simulink library "INT_CoETS_TSEACo"  (R2016b)
settings: Solver=VariableStepAuto  StartTime=0.0  StopTime=10.0  RelTol=1e-3
settings Model: Creator=xuxingpei  LastModifiedBy=xuxingpei

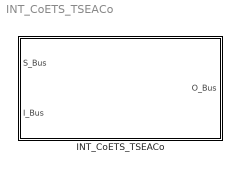
== system INT_CoETS_TSEACo ==
  INT_CoETS_TSEACo : Subsystem

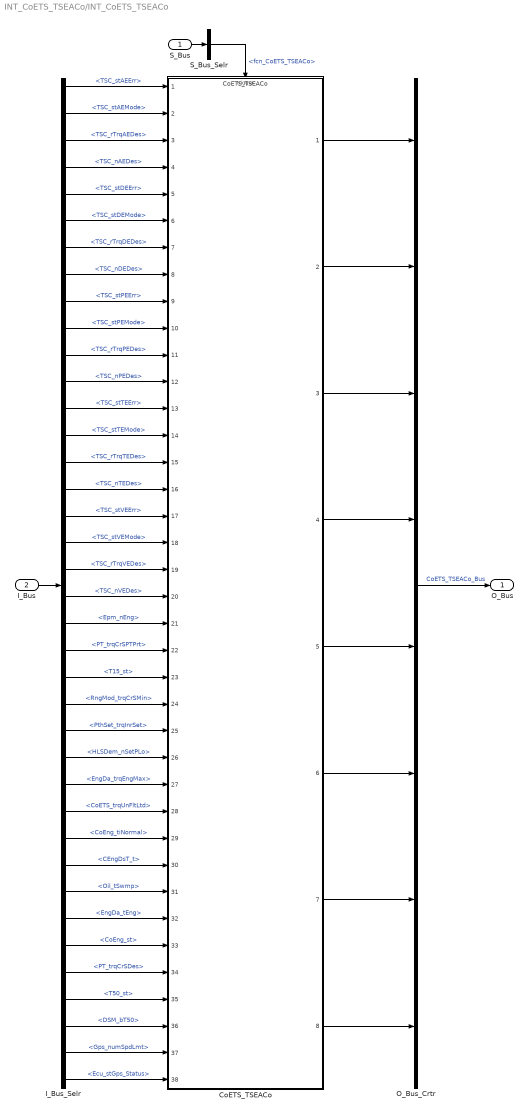
== system INT_CoETS_TSEACo/INT_CoETS_TSEACo ==
  S_Bus : Inport
  I_Bus : Inport  Port=2
  CoETS_TSEACo : ModelReference  ModelNameDialog=CoETS_TSEACo  SimulationMode=Normal  ModelReferenceVersion=1.404  TriggerPortName=function  TriggerPortTriggerType=function-call  TriggerPortStatesWhenEnabling=held
  I_Bus_Selr : BusSelector  OutputSignals=TSC_stAEErr,TSC_stAEMode,TSC_rTrqAEDes,TSC_nAEDes,TSC_stDEErr,TSC_stDEMode,TSC_rTrqDEDes,TSC_nDEDes,TSC_stPEErr,TSC_stPEMode,TSC_rTrqPEDes,TSC_nPEDes,TSC_stTEErr,TSC_stTEMode,TSC_rTrqTEDes,TSC_nTEDes,TSC_stVEErr,TSC_stVEMode,TSC_rTrqVEDes,TSC_nVEDes,Epm_nEng,PT_trqCrSPTPrt,T15_st,RngMod_trqCrSMin,PthSet_trqInrSet,HLSDem_nSetPLo,EngDa_trqEngMax,CoETS_trqUnFltLtd,CoEng_tiNormal,CEngDsT_t,Oil_tSwmp,EngDa_tEng,CoEng_st,PT_trqCrSDes,T50_st,DSM_bT50,Gps_numSpdLmt,Ecu_stGps_Status
  O_Bus_Crtr : BusCreator  Inputs=8
  S_Bus_Selr : BusSelector  OutputSignals=fcn_CoETS_TSEACo
  O_Bus : Outport
  wires:
  S_Bus_Selr/1 -> CoETS_TSEACo/Trigger  "<fcn_CoETS_TSEACo>"
  S_Bus/1 -> S_Bus_Selr/1
  I_Bus/1 -> I_Bus_Selr/1
  I_Bus_Selr/1 -> CoETS_TSEACo/1  "<TSC_stAEErr>"
  I_Bus_Selr/2 -> CoETS_TSEACo/2  "<TSC_stAEMode>"
  I_Bus_Selr/3 -> CoETS_TSEACo/3  "<TSC_rTrqAEDes>"
  I_Bus_Selr/4 -> CoETS_TSEACo/4  "<TSC_nAEDes>"
  I_Bus_Selr/5 -> CoETS_TSEACo/5  "<TSC_stDEErr>"
  I_Bus_Selr/6 -> CoETS_TSEACo/6  "<TSC_stDEMode>"
  I_Bus_Selr/7 -> CoETS_TSEACo/7  "<TSC_rTrqDEDes>"
  I_Bus_Selr/8 -> CoETS_TSEACo/8  "<TSC_nDEDes>"
  I_Bus_Selr/9 -> CoETS_TSEACo/9  "<TSC_stPEErr>"
  I_Bus_Selr/10 -> CoETS_TSEACo/10  "<TSC_stPEMode>"
  I_Bus_Selr/11 -> CoETS_TSEACo/11  "<TSC_rTrqPEDes>"
  I_Bus_Selr/12 -> CoETS_TSEACo/12  "<TSC_nPEDes>"
  I_Bus_Selr/13 -> CoETS_TSEACo/13  "<TSC_stTEErr>"
  I_Bus_Selr/14 -> CoETS_TSEACo/14  "<TSC_stTEMode>"
  I_Bus_Selr/15 -> CoETS_TSEACo/15  "<TSC_rTrqTEDes>"
  I_Bus_Selr/16 -> CoETS_TSEACo/16  "<TSC_nTEDes>"
  I_Bus_Selr/17 -> CoETS_TSEACo/17  "<TSC_stVEErr>"
  I_Bus_Selr/18 -> CoETS_TSEACo/18  "<TSC_stVEMode>"
  I_Bus_Selr/19 -> CoETS_TSEACo/19  "<TSC_rTrqVEDes>"
  I_Bus_Selr/20 -> CoETS_TSEACo/20  "<TSC_nVEDes>"
  I_Bus_Selr/21 -> CoETS_TSEACo/21  "<Epm_nEng>"
  I_Bus_Selr/22 -> CoETS_TSEACo/22  "<PT_trqCrSPTPrt>"
  I_Bus_Selr/23 -> CoETS_TSEACo/23  "<T15_st>"
  I_Bus_Selr/24 -> CoETS_TSEACo/24  "<RngMod_trqCrSMin>"
  I_Bus_Selr/25 -> CoETS_TSEACo/25  "<PthSet_trqInrSet>"
  I_Bus_Selr/26 -> CoETS_TSEACo/26  "<HLSDem_nSetPLo>"
  I_Bus_Selr/27 -> CoETS_TSEACo/27  "<EngDa_trqEngMax>"
  I_Bus_Selr/28 -> CoETS_TSEACo/28  "<CoETS_trqUnFltLtd>"
  I_Bus_Selr/29 -> CoETS_TSEACo/29  "<CoEng_tiNormal>"
  I_Bus_Selr/30 -> CoETS_TSEACo/30  "<CEngDsT_t>"
  I_Bus_Selr/31 -> CoETS_TSEACo/31  "<Oil_tSwmp>"
  I_Bus_Selr/32 -> CoETS_TSEACo/32  "<EngDa_tEng>"
  I_Bus_Selr/33 -> CoETS_TSEACo/33  "<CoEng_st>"
  I_Bus_Selr/34 -> CoETS_TSEACo/34  "<PT_trqCrSDes>"
  I_Bus_Selr/35 -> CoETS_TSEACo/35  "<T50_st>"
  I_Bus_Selr/36 -> CoETS_TSEACo/36  "<DSM_bT50>"
  I_Bus_Selr/37 -> CoETS_TSEACo/37  "<Gps_numSpdLmt>"
  I_Bus_Selr/38 -> CoETS_TSEACo/38  "<Ecu_stGps_Status>"
  O_Bus_Crtr/1 -> O_Bus/1  "CoETS_TSEACo_Bus"
  CoETS_TSEACo/1 -> O_Bus_Crtr/1
  CoETS_TSEACo/2 -> O_Bus_Crtr/2
  CoETS_TSEACo/3 -> O_Bus_Crtr/3
  CoETS_TSEACo/4 -> O_Bus_Crtr/4
  CoETS_TSEACo/5 -> O_Bus_Crtr/5
  CoETS_TSEACo/6 -> O_Bus_Crtr/6
  CoETS_TSEACo/7 -> O_Bus_Crtr/7
  CoETS_TSEACo/8 -> O_Bus_Crtr/8
